simulink model "QAM"  (R2023b)
settings: Solver=VariableStepAuto  StartTime=0.0  StopTime=50  RelTol=1e-3
libraries: commrflib2 x1, commrandsrc3 x1
settings Model: Creator=HP  LastModifiedBy=HP

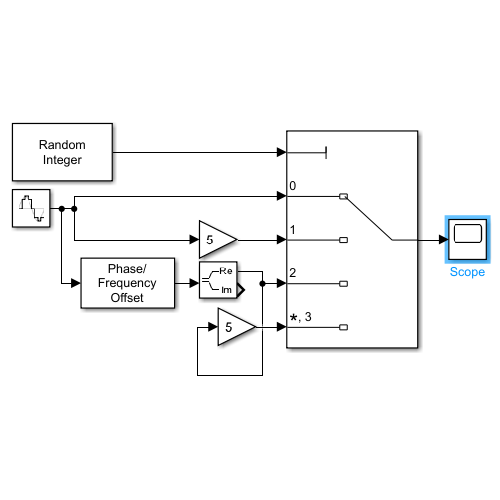
[thumbnail: Simulink's stored preview of the top-level diagram]
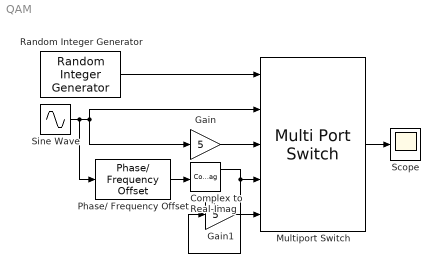
== system QAM ==
  Complex to Real-Imag : ComplexToRealImag
  Gain : Gain  Gain=5
  Gain1 : Gain  Gain=5
  Multiport Switch : MultiPortSwitch  DataPortOrder=Zero-based contiguous  Inputs=4  zeroidx=on  SaturateOnIntegerOverflow=off  InputSameDT=off
  Phase/ Frequency Offset : commrflib2/Phase// Frequency Offset  phaseOffset=180  freqPort=off  freqOffset=0
  Random Integer Generator : commrandsrc3/Random Integer Generator  SetSize=3  SeedSource=Auto  Seed=0  SampleTime=0.5  SamplesPerFrame=1  OutputDataType=double  SimulateUsing=Interpreted execution
  Scope : Scope
  Sine Wave : Sin  Frequency=2*pi  SampleTime=0.01
  wires:
  Random Integer Generator/1 -> Multiport Switch/1
  Sine Wave/1 -> Phase/ Frequency Offset/1, Gain/1, Multiport Switch/2
  Gain/1 -> Multiport Switch/3
  Gain1/1 -> Multiport Switch/5
  Multiport Switch/1 -> Scope/1
  Phase/ Frequency Offset/1 -> Complex to Real-Imag/1
  Complex to Real-Imag/1 -> Gain1/1, Multiport Switch/4
